simulink model "blocks"  (R2019a)
settings: Solver=VariableStepAuto  StartTime=0.0  StopTime=10.0  RelTol=1e-3
settings Model: Creator=adeye  LastModifiedBy=adeye

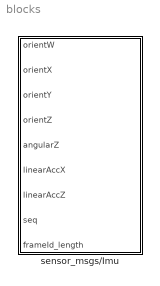
== system blocks ==
  sensor_msgs/Imu : Subsystem  mask{topic='/imu_raw', message_type='sensor_msgs/Imu', port=9090, timeout=2}
      mask prompts: topic "Topic name"; message_type "Message type"; timeout "Timeout (s)"

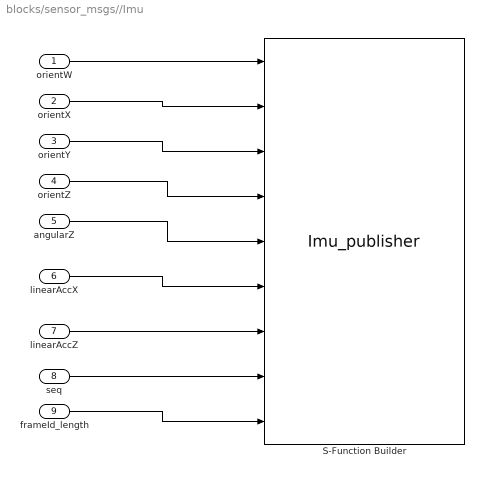
== system blocks/sensor_msgs//Imu ==
  orientW : Inport
  orientX : Inport  Port=2
  orientY : Inport  Port=3
  orientZ : Inport  Port=4
  angularZ : Inport  Port=5
  linearAccX : Inport  Port=6
  linearAccZ : Inport  Port=7
  seq : Inport  Port=8
  frameId_length : Inport  Port=9
  S-Function Builder : S-Function  InitFcn=try, set_param(gcb,'FunctionName','Imu_publisher'), end  FunctionName=Imu_publisher  Parameters=int8(topic),int8(message_type),port,timeout  SFunctionModules=Imu_publisher_wrapper rosbridge_functions  SFunctionDeploymentMode=off  EnableBusSupport=off  mask(S-Function Builder){}
      mask help: Simulink:masks:SFunctionBuilder_MD
      mask init:
      | val = [[.9  0.75 0.75 1 1 .9 .9 1]',[1 1 0.75 0.75 .9 .9 1 .9]'];try , sys = get_param(gcb,'SfunBuilderFcnName');if isempty(sys), sys = get_param(gcb,'FunctionName'); end,catch, sys = get_param(gcb,'FunctionName'); end
      settings: CopyFcn=set_param(gcbh,'LinkStatus','none')  PreSaveFcn=try, set_param(gcb,'FunctionName','Imu_publisher'), end  OpenFcn=sfunctionwizard(gcbh)
      mask Display: plot(val(:,1),val(:,2)),disp(sys), port_label('input',1,'orientW'), port_label('input',2,'orientX'), port_label('input',3,'orientY'), port_label('input',4,'orientZ'), port_label('input',5,'angularZ'), port_label('input',6,'linearAccX'), port_label('input',7,'linearAccZ'), port_label('input',8,'seq'), port_label('input',9,'frameId_length')
  wires:
  orientW/1 -> S-Function Builder/1
  linearAccZ/1 -> S-Function Builder/7
  seq/1 -> S-Function Builder/8
  orientX/1 -> S-Function Builder/2
  orientY/1 -> S-Function Builder/3
  linearAccX/1 -> S-Function Builder/6
  frameId_length/1 -> S-Function Builder/9
  orientZ/1 -> S-Function Builder/4
  angularZ/1 -> S-Function Builder/5
